simulink subsystem "cycling_automata"  (R2022a)
settings: Solver=VariableStepAuto  StartTime=0.0  StopTime=10.0  RelTol=1e-3
settings Model: Creator=mateu  LastModifiedBy=mateu

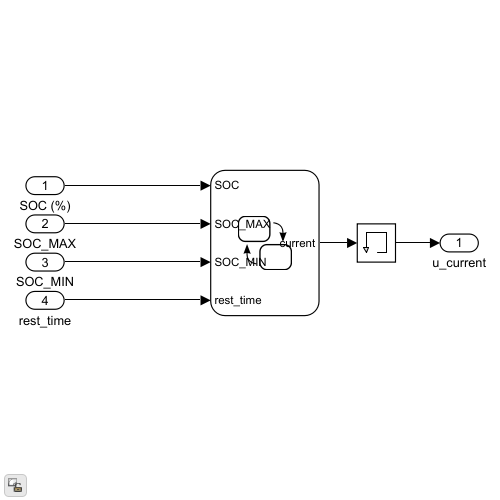
[thumbnail: Simulink's stored preview of the top-level diagram]
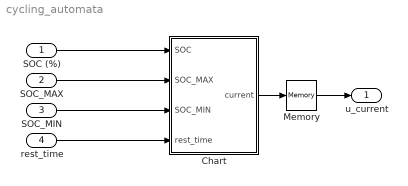
== system cycling_automata ==
  SOC (%) : Inport
  SOC_MAX : Inport  Port=2
  SOC_MIN : Inport  Port=3
  rest_time : Inport  Port=4
  Chart : Stateflow chart  TreatAsAtomicUnit=on
      settings: PortSchema="{\"entries\":[{\"content\":{\"sides\":[{\"content\":{\"connectorIds\":[\"In2\",\"In3\",\"In4\",\"In1\"]},\"type\":\"ConnectorPlacement.EquallySpacedRectSide\",\"uuid\":\"b79e6304-446b-4da0-b841-6a7e0125cfd5\"},{\"content\":{\"connectorIds\":[\"Out1\"],\"side\":\"RIGHT\"},\"type\":\"ConnectorPlacement.EquallySpacedRectSide\",\"uuid\":\"907ab61a-1d0a-45c7-8983-f54ad408e9d5\"},{\"content\":{\"connectorIds\":[],\"side\":\"TOP\"},\"type\":\"ConnectorPlacement.EquallySpacedRectSide\",\"uuid\":\"544cfd83-6b45-4625-b149-12de8a160085\"}]},\"type\":\"ConnectorPlacement.EquallySpacedConnector\",\"uuid\":\"2fa71fdc-98f6-47db-8b29-348eadeade42\"}],\"packageUris\":[\"http://schema.mathworks.com/mf0/Connector/R2020b\"],\"version\":\"1.0\"}"
  Memory : Memory
  u_current : Outport
  wires:
  rest_time/1 -> Chart/1(rest_time)
  Chart/1(current) -> Memory/1
  SOC (%)/1 -> Chart/2(SOC)
  Memory/1 -> u_current/1
  SOC_MAX/1 -> Chart/3(SOC_MAX)
  SOC_MIN/1 -> Chart/4(SOC_MIN)

== stateflow chart cycling_automata/Chart ==
  settings: executeAtInitialization=1
  state Descarga
    current=-40;
  state Repouso
    current=0;
  state Recarga
    current=60;
  (junction 23) -> Descarga [order 1] : [SOC>=SOC_MAX]
  Descarga -> Recarga : [SOC<=SOC_MIN]
  (default) -> Repouso
  Repouso -> (junction 23) : [after(rest_time,sec)]
  (junction 23) -> Recarga [order 2]
  Recarga -> Repouso : [SOC>=SOC_MAX]
  data: rest_time input; current output; SOC input; SOC_MAX input; SOC_MIN input
